simulink model "example_Storage_type5conf"  (R2016b)
settings: Solver=ode45  StartTime=0.0  StopTime=3*3600-2  MaxStep=300  RelTol=1e-3  EnableMultiTasking=on
undefined symbols (not defined in the file): path_carnot
libraries: carnot x18, simulink x5
settings Model: DEBUGGLOBALLEVEL=DEBUGLEVEL  DEBUGMAXTOTALWARNINGS=100  DEBUGMAXCONSECUTIVEWARNINGS=100  DEBUGWRITETOFILE=0  DEBUGFILENAME='error.txt'  Creator=drhf  LastModifiedBy=drhf
settings DataIOCC: LimitDataPoints=on  SaveFormat=Array
settings OptimizationCC: ExpressionDepthLimit=2147483647  LifeSpan=inf
settings DebuggingCC: UnderspecifiedInitializationDetection=Classic  MergeDetectMultiDrivingBlocksExec=none  SolverPrmCheckMsg=warning  StateNameClashWarn=warning  SFUnexpectedBacktrackingDiag=warning  SFNoUnconditionalDefaultTransitionDiag=warning  SFExecutionAtInitializationDiag=none
settings HardwareCC: ProdBitPerPointer=32  ProdBitPerSizeT=32  ProdBitPerPtrDiffT=32  ProdLargestAtomicFloat=None  ProdIntDivRoundTo=Undefined  ProdEndianess=Unspecified  ProdWordSize=32  ProdHWDeviceType=32-bit Generic
settings ModelReferenceCC: PropagateSignalLabelsOutOfModel=off
settings GRTTargetCC: TargetLangStandard=C89/C90 (ANSI)  GeneratePreprocessorConditionals=Disable all  CombineOutputUpdateFcns=off  GRTInterface=on
settings ConfigComp: CovMetricSettings=dw  CovHtmlReporting=on  CovSaveCumulativeToWorkspaceVar=on  CovSaveSingleToWorkspaceVar=on  CovExternalEMLEnable=off

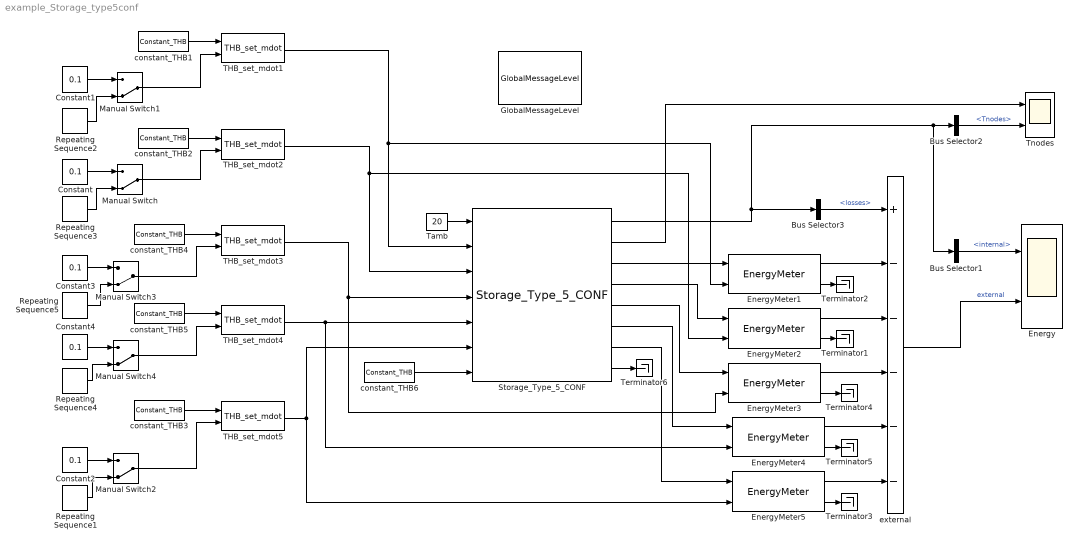
== system example_Storage_type5conf ==
  Bus Selector1 : BusSelector  OutputSignals=energy.internal
  Bus Selector2 : BusSelector  OutputSignals=Tnodes
  Bus Selector3 : BusSelector  OutputSignals=energy.losses
  Constant{,1..4} (5 alike) : Constant  Value=0.1
  Energy : Scope  NumInputPorts=2
  EnergyMeter{1..5} (5 alike) : carnot/Control/EnergyMeter
  GlobalMessageLevel : carnot/Toolbox/GlobalMessageLevel  GLOBALLOCAL=global  DEBUGLEVEL=DEBUGLEVEL  MAXTOTALWARNINGS=100  MAXCONSECUTIVEWARNINGS=100  WRITETOFILE=0  FILENAME='error.txt'
  Manual Switch{,1..4} (5 alike) : ManualSwitch  CurrentSetting=0
  Repeating Sequence1 : simulink/Sources/Repeating Sequence  rep_seq_t=[ 0 3600 3600+eps(3600) 7200 7200+eps(7200) 10800]  rep_seq_y=[ 0.12 0.12 0.11+0*eps(3600) 0.11 0.05+0*eps(7200) 0.05]
  Repeating Sequence2 : simulink/Sources/Repeating Sequence  rep_seq_t=[ 0 3600 3600+eps(3600) 7200 7200+eps(7200) 10440 10440+eps(10440) 11160]  rep_seq_y=[ 0 0 0.05+0*eps(3600) 0.05 0.2+0*eps(7200) 0.2 0+0*eps(10440) 0]
  Repeating Sequence3 : simulink/Sources/Repeating Sequence  rep_seq_t=[ 0 3600 3600+eps(3600) 7200 7200+eps(7200) 10800]  rep_seq_y=[ 0 0 0.1+0*eps(3600) 0.1 0.15+0*eps(7200) 0.15]
  Repeating Sequence4 : simulink/Sources/Repeating Sequence  rep_seq_t=[ 0 3600 3600+eps(3600) 7200 7200+eps(7200) 10800]  rep_seq_y=[ 0.11 0.11 0.1+0*eps(3600) 0.1 0.11+0*eps(7200) 0.11]
  Repeating Sequence5 : simulink/Sources/Repeating Sequence  rep_seq_t=[ 0 3600 3600+eps(3600) 7200 7200+eps(7200) 10800]  rep_seq_y=[ 0.11 0.11 0.1+0*eps(3600) 0.1 0.11+0*eps(7200) 0.11]
  Storage_Type_5_CONF : carnot/Storage/Thermal/Storage_Type_5_CONF  t0=[10:5:55]  tini=[10 12.3684210526316 14.7368421052632 17.1052631578947 19.4736842105263 21.8421052631579 24.2105263157895 26.5789473684211 28.9473684210526 31.3157894736842 33.6842105263158 36.0526315789474 38.4210526315789 40.7894736842105 43.1578947368421 45.5263157894737 47.8947368421053 50.2631578947368 52.6315789473684 55]  hgt=1.8108  mpts=[1 3 5 7 9 11 13 15 17 19]  PathName=fullfile(path_carnot('libsl'),'Storage','Thermal','Storage_Type_5_CONF','parameter_set')  FileName='StorageType5_800_L.mat'  userPath=off  userParam=off  uwall=1  ubot=1  utop=1  axcond=1  volume=0.8  dia=0.75  standing=standing cylinder  nodes=20  mpoints=10  Tsensor=[0.2 0.5 0.7]  pipe3inlet=1  pipe3outlet=0.6  pipe3dia=0.05  pipe1inlet=0.55  pipe1outlet=0.45  pipe1dia=0.05  hx1inlet=0.4  hx1outlet=0  hx1dia=0.03  hx1uac=200  hx1uam=0.15  hx1uat=0.6  hx1dplin=20  hx1dpqua=20  pipe2inlet=0.45  pipe2outlet=0.55  pipe2dia=0.05  hx2inlet=0  hx2outlet=1  hx2dia=0.025  hx2uac=450  hx2uam=0.4  hx2uat=0.8  hx2dplin=200  hx2dpqua=200  hx3inlet=0.9  hx3outlet=1  hx3dia=0.01  hx3uac=100  hx3uam=0  hx3uat=0  hx3dplin=10  hx3dpqua=10
  THB_set_mdot{1..5} (5 alike) : carnot/Source/Simple/THB_set_mdot
  Tamb : Constant  Value=20
  Terminator{1..6} (6 alike) : Terminator
  Tnodes : Scope  NumInputPorts=2
  constant_THB1 : carnot/Source/Simple/Constant_THB  t=15  mdot=0*100/3600  p=1e5  mID=Full Pressure Drop with Static Height  fluid=Water  mix=0  mix2=0  mix3=0  dia=0.02  hgt=0
  constant_THB2 : carnot/Source/Simple/Constant_THB  t=60  mdot=100/3600  p=1e5  mID=Full Pressure Drop with Static Height  fluid=Water  mix=0  mix2=0  mix3=0  dia=0.02  hgt=0
  constant_THB3 : carnot/Source/Simple/Constant_THB  t=40  mdot=100/3600  p=1e5  mID=Full Pressure Drop with Static Height  fluid=Water  mix=0  mix2=0  mix3=0  dia=0.02  hgt=0
  constant_THB4 : carnot/Source/Simple/Constant_THB  t=30  mdot=100/3600  p=1e5  mID=Full Pressure Drop with Static Height  fluid=Water  mix=0  mix2=0  mix3=0  dia=0.02  hgt=0
  constant_THB5 : carnot/Source/Simple/Constant_THB  t=40  mdot=100/3600  p=1e5  mID=Full Pressure Drop with Static Height  fluid=Water  mix=0  mix2=0  mix3=0  dia=0.02  hgt=0
  constant_THB6 : carnot/Source/Simple/Constant_THB  t=40  mdot=0  p=1e5  mID=Full Pressure Drop with Static Height  fluid=Water  mix=0  mix2=0  mix3=0  dia=0.02  hgt=0
  external : Sum  Inputs=+-----
  wires:
  Tamb/1 -> Storage_Type_5_CONF/1
  THB_set_mdot1/1 -> Storage_Type_5_CONF/2, EnergyMeter1/2
  THB_set_mdot2/1 -> Storage_Type_5_CONF/3, EnergyMeter2/2
  EnergyMeter2/2 -> Terminator1/1
  constant_THB1/1 -> THB_set_mdot1/1
  constant_THB2/1 -> THB_set_mdot2/1
  Manual Switch1/1 -> THB_set_mdot1/2
  Manual Switch/1 -> THB_set_mdot2/2
  Constant/1 -> Manual Switch/1
  Repeating Sequence3/1 -> Manual Switch/2
  Constant1/1 -> Manual Switch1/1
  Repeating Sequence2/1 -> Manual Switch1/2
  EnergyMeter1/2 -> Terminator2/1
  external/1 -> Energy/2  "external"
  EnergyMeter2/1 -> external/3
  EnergyMeter1/1 -> external/2
  constant_THB3/1 -> THB_set_mdot5/1
  Manual Switch2/1 -> THB_set_mdot5/2
  Constant2/1 -> Manual Switch2/1
  Repeating Sequence1/1 -> Manual Switch2/2
  THB_set_mdot5/1 -> Storage_Type_5_CONF/6, EnergyMeter5/2
  EnergyMeter5/2 -> Terminator3/1
  constant_THB4/1 -> THB_set_mdot3/1
  Manual Switch3/1 -> THB_set_mdot3/2
  Constant3/1 -> Manual Switch3/1
  Repeating Sequence5/1 -> Manual Switch3/2
  THB_set_mdot3/1 -> Storage_Type_5_CONF/4, EnergyMeter3/2
  EnergyMeter3/2 -> Terminator4/1
  EnergyMeter3/1 -> external/4
  constant_THB5/1 -> THB_set_mdot4/1
  Manual Switch4/1 -> THB_set_mdot4/2
  Constant4/1 -> Manual Switch4/1
  Repeating Sequence4/1 -> Manual Switch4/2
  THB_set_mdot4/1 -> Storage_Type_5_CONF/5, EnergyMeter4/2
  EnergyMeter4/2 -> Terminator5/1
  EnergyMeter4/1 -> external/5
  EnergyMeter5/1 -> external/6
  Storage_Type_5_CONF/1 -> Bus Selector2/1, Bus Selector1/1, Bus Selector3/1
  Bus Selector1/1 -> Energy/1  "<internal>"
  Bus Selector2/1 -> Tnodes/2  "<Tnodes>"
  Storage_Type_5_CONF/2 -> Tnodes/1
  constant_THB6/1 -> Storage_Type_5_CONF/7
  Bus Selector3/1 -> external/1  "<losses>"
  Storage_Type_5_CONF/3 -> EnergyMeter1/1
  Storage_Type_5_CONF/4 -> EnergyMeter2/1
  Storage_Type_5_CONF/5 -> EnergyMeter3/1
  Storage_Type_5_CONF/6 -> EnergyMeter4/1
  Storage_Type_5_CONF/7 -> EnergyMeter5/1
  Storage_Type_5_CONF/8 -> Terminator6/1
